simulink model "Boeing787_NewMission_ElectricalThermal"  (R2016a)
settings: Solver=ode23tb  SolverMode=SingleTasking  StartTime=0.0  StopTime=18000  RelTol=1e-3
InitFcn:
  | load('SampleOutput.mat')
  | 
  | load('SampleFuelBurn.mat')
StartFcn:
  | tic
StopFcn:
  | ttt = toc
  | tend = eval(get_param(bdroot,'StopTime'));
  | disp(['Total Simulation Time (s) = ' num2str(ttt) 's']);
  | RTR =  ttt/tend
  | disp(['Simulation Speed is ' num2str(tend/ttt) 'x faster than real-time']);
undefined symbols (not defined in the file): CurrentMission, FuelBurn, seed
libraries: PowerFlowLib x18, simulink x12, powerlib_meascontrol x1
(part 2 of 17)

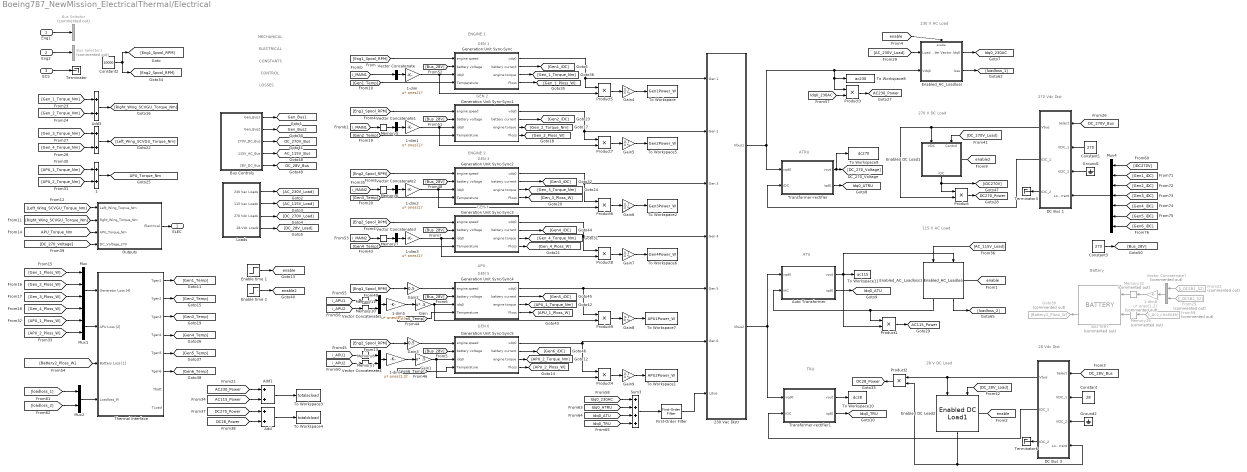
== system Boeing787_NewMission_ElectricalThermal/Electrical ==
  note: ATRU
  note: TRU
  note: 230 V AC Load
  note: 270 Vdc Dist
  note: 28 Vdc Dist
  note: 270 V DC Load
  note: CONSTANTS
  note: CONTROL
  note: LOSSES
  note: MECHANICAL
  note: ELECTRICAL
  note: ATU
  note: 115 V AC Load
  note: 28 V DC Load
  note: Battery
  note: GEN 1
  note: ENGINE 1
  note: GEN 2
  note: GEN 3
  note: ENGINE 2
  note: GEN 4
  note: GEN 5
  note: APU
  note: GEN 6
  Eng1 : Inport
  Eng2 : Inport  Port=2
  ECS : Inport  Port=3
  " " : Sum
  " 1" : Sum
  1-dim{,1..3} (4 alike) : Gain  Gain=ones(1)'  Multiplication=Matrix(u*K)
  1-dim4 : Gain  Gain=ones(1,2)'  Multiplication=Matrix(u*K)
  1-dim5 : Gain  Gain=ones(1,2)'  Multiplication=Matrix(u*K)
  1-dim8 : Gain  Commented=on  Gain=ones(1,2)'  Multiplication=Matrix(u*K)
  230 Vac Distr : Subsystem
  Add : Sum
  Add1 : Sum
  Add3 : Sum
  Auto Transformer : Subsystem  AncestorBlock=PowerFlowLib/Energy & Power Systems/Electrical/Systems/Transformer-rectifier  mask{pu=1}
      mask prompts: pu "Voltage Regulation Level (p.u.)"
      mask Display:
      | image('ATU.png')
      | % Define Inputs
      | port_label('input',1,'{\bf V_d_q_0}','Texmode','on')
      | port_label('input',2,'{\bf i_{dq0}}','Texmode','on')
      | 
      | % Define Outputs
      | port_label('output',1,'{\bf V_d_q_0}','Texmode','on')
      | port_label('output',2,'{\bf I_d_q_0}','Texmode','on')
      | 
      | 
      | % % Define Inputs
      | % port_label('input',1,'{\bf Line Voltage}','Texmode','on')
      | % port_label('input',2,'{\bf Line Voltage}','Texmode','on')
      | %
      | % % Define Outputs
      | % port_label('output',1,'{\bf Line Voltage}','Texmode','on')
      | % port_label('output',2,'{\bf Line Voltage}','Texmode','on')
  BATTERY : PowerFlowLib/Energy & Power Systems/Electrical/Battery/BATTERY  Commented=on  NO_CELLS=9  NO_MODULES=10  INITIAL_SOC=1
  Bus Selector : BusSelector  Commented=on  OutputSignals=Spools.HPSpoolSpeed_rpm
  Bus Selector1 : BusSelector  Commented=on  OutputSignals=Spools.HPSpoolSpeed_rpm
  Bus Controls : Subsystem  mask{BUS1=Generator 1, BUS2=Generator 2, MBUS1=Generator Bus 1, ACTBUS1=Generator Bus 1, MBUS2=Generator Bus 2, ACTBUS2=Generator Bus 2, IDCBUS1=Battery 1, IDCBUS2=Battery 2}
      mask prompts: BUS1 "Source for Bus 1"; BUS2 "Source for Bus 2"; MBUS1 "Load on Main Bus 1 drawn from"; ACTBUS1 "Load on AC Transfer Bus 1 drawn from"; MBUS2 "Load on Main Bus 2 drawn from"; ACTBUS2 "Load on AC Transfer Bus 2 drawn from"; IDCBUS1 "Source for DC Service Bus 1"; IDCBUS2 "Source for DC Service Bus 2"
      mask help:
      | Specify the source from which different buses receive power. There are
      | 1. Two Generator buses (Bus 1-2)
      | 2. Two AC Main buses (Main Bus 1-2))
      | 3. Two AC Transfer buses and (AC Transfer Bus 1-2)
      | 4. Two DC Intermediate buses (DC Intermediate Bus 1-2)
      mask init:
      | switch BUS1
      |     case 1
      |         BUS1CONTROL = 1;
      |     case 2
      |         BUS1CONTROL = 2;
      |     case 3
      |         BUS1CONTROL = 3;
      |     case 4
      |         BUS1CONTROL = 4;
      | end
      | 
      | switch BUS2
      |     case 1
      |         BUS2CONTROL = 1;
      |     case 2
      |         BUS2CONTROL = 2;
      |     case 3
      |         BUS2CONTROL = 3;
      |     case 4
      |         BUS2CONTROL = 4;
      | end
      | 
      | switch MBUS1
      |     case 1
      |         MBUS1CONTROL = 1;
      |     case 2
      |         MBUS1CONTROL = 2;
      | end
      | 
      | switch ACTBUS1
      |     case 1
      |         ACTBUS1CONTROL = 1;
      |     case 2
      |         ACTBUS1CONTROL = 2;
      | end
      | 
      | switch MBUS2
      |     case 1
      |         MBUS2CONTROL = 1;
      |     case 2
      |         MBUS2CONTROL = 2;
      | end
      | 
      | switch ACTBUS2
      |     case 1
      |         ACTBUS2CONTROL = 1;
      |     case 2
      |         ACTBUS2CONTROL = 2;
      | end
      | 
      | switch IDCBUS1
      |     case 1
      |         IDCBUS1CONTROL = 1;
      |     case 2
      |         IDCBUS1CONTROL = 2;
      | end
      | 
      | switch IDCBUS2
      |     case 1
      |         IDCBUS2CONTROL = 1;
      |     case 2
      |         IDCBUS2CONTROL = 2;
      | end
      mask TypeOptions BUS1: Generator 1  | APU  | GND | AUX SUPPLY
      mask TypeOptions BUS2: Generator 2  | APU  | GND | AUX SUPPLY
      mask TypeOptions MBUS1: Generator Bus 1 | Generator Bus 2
      mask TypeOptions ACTBUS1: Generator Bus 1 | Generator Bus 2
      mask TypeOptions MBUS2: Generator Bus 1 | Generator Bus 2
      mask TypeOptions ACTBUS2: Generator Bus 1 | Generator Bus 2
      mask TypeOptions IDCBUS1: Battery 1 | Battery 2
      mask TypeOptions IDCBUS2: Battery 1 | Battery 2
  Constant : Constant  Value=28
  Constant1 : Constant  Value=270
  Constant2 : Constant  Value=10000
  Constant3 : Constant  Value=270
  DC Bus 1 : Subsystem  mask(DC Service Bus){}
      mask help: Service Bus
  DC Bus 3 : Subsystem  mask(DC Service Bus){}
      mask help: Service Bus
  Enable time 1 : Step  Time=100  SampleTime=0
  Enable time 2 : Step  Time=105  SampleTime=0
  Enabled DC Load1 : Subsystem  AncestorBlock="PowerFlowLib/Energy & Power Systems/Electrical/Loads/Enabled  DC Load1"
      mask help: Enabled DC Load System.
      mask Display:
      | image(imread('DCloads.png'))
      | 
      | port_label('input',1,'{\bf V_D_C}','TexMode','on')
      | port_label('input',2,'{\bf Load}','TexMode','on')
      | port_label('Enable','{\bf switch}','Texmode','on')
      | 
      | port_label('output',1,'{\bf I_D_C}','TexMode','on')
  Enabled DC Load2 : PowerFlowLib/Energy & Power Systems/Electrical/Loads/Enabled  DC Load1
  Enabled_AC_Loadloss : Subsystem  AncestorBlock=PowerFlowLib/Energy & Power Systems/Electrical/Loads/Enabled_AC_Loadloss  mask(AC Loads){P=500, PF=0.85, ILRMS=0, R=10000, X=10000}
      mask prompts: P "Real Power (W)"; PF "Power factor (Range: 0 -1) : Prefix '-' sign for Cap loads"; ILRMS "Current Loading"; R "Resistance (Ohms)"; X "Reactance (Ohms)"
      mask help:
      | Enabled AC Load System.
      | Note:
      | Load Master Vector input is 1x3 matrix representing (P[W] Q[Var] I[A])
      | Extra load can be input in the boxes below and will be added with the Load Master Vector.
      mask Help: eval('open(''AC Loads_help.html'')');
      mask Callback PF:
      | blk = gcb;
      | PF    = str2num(get_param(blk,'PF'));
      | 
      | if ((PF>1) | (PF<-1))
      |    g = warndlg('Power factor magnitude should be between 0 and 1 . Reverting to default value 1','Error1','CreateMode');
      |    set_param(blk,'PF','1');
      |    open_system(blk,'mask');
      | end
      | 
      | clear g PF blk
      mask Callback X:
      | blk = gcb;
      | value1 = str2num(get_param(blk,'R'));
      | value2 = str2num(get_param(blk,'X'));
      | % eff    = str2num(get_param(blk,'E'));
      | 
      | if (value1==0) && (value2==0)
      |   h = warndlg('Both R and X cannot be 0. Reverting to default values','Error','CreateMode');
      |   set_param(blk,'R','10000');
      |   set_param(blk,'X','10000');
      | %   if ishandle(h)
      | %       close(h)
      |   open_system(blk,'mask');
      | end
      | 
      | % if ((eff>1) | (eff<0))
      | %    g = warndlg('Efficiency should be between 0 and 1 . Reverting to default value 1','Error1','CreateMode');
      | %    set_param(blk,'E','1');
      | %    open_system(blk,'mask');
      | % end
      | 
      | clear h eff blk value1 value2
      mask Display:
      | %image(imread('ACload.png'))
      | 
      | % port_label('input',1,'{\bf EXT LOAD VECTOR}','TexMode','on')
      | % port_label('input',2,'{\bf Vdq0}','TexMode','on')
      | %
      | % port_label('output',1,'{\bf Idq0}','TexMode','on')
      | % port_label('output',2,'{\bf PLOSS}','TexMode','on')
      | 
      | image(imread('ACloads.png'))
      | 
      | port_label('input',1,'{\bf Load}','TexMode','on')
      | port_label('input',2,'{\bf V_d_q_0}','TexMode','on')
      | port_label('Enable','{\bf switch}','Texmode','on')
      | 
      | port_label('output',1,'{\bf I_d_q_0}','TexMode','on')
      | port_label('output',2,'{\bf P_l_o_s_s}','TexMode','on')
  Enabled_AC_Loadloss1 : PowerFlowLib/Energy & Power Systems/Electrical/Loads/Enabled_AC_Loadloss  P=500  PF=0.85  ILRMS=0  R=10000  X=10000
  First-Order Filter : powerlib_meascontrol/Filters/First-Order Filter  FilterType=Lowpass  Tc=10e-1  Ts=0  Initialize=on  Vac_Init=[0, 0, 60]  Vdc_Init=0  PlotResponse=off  FreqRange="[0,  200,  1]"
  From22 : From  Commented=on  GotoTag=i_DCSB1_S2
  From25 : From  Commented=on  GotoTag=i_DCSB2_S2
  From59 : From  Commented=on  GotoTag=i_DC2_CHARGER
  Gain : Gain  Gain=.5  Multiplication=Matrix(u*K)
  Gain1 : Gain  Gain=.5  Multiplication=Matrix(u*K)
  Gain2 : Gain  Gain=0.5
  Gain3 : Gain  Gain=0.5
  Gain{4..9} (6 alike) : Gain  Gain=[1 1 1]  Multiplication=Matrix(K*u) (u vector)
  Generation Unit Sync-Sync : Subsystem  AncestorBlock=PowerFlowLib/Energy & Power Systems/Electrical/Systems/Generation Unit Sync-Sync  mask{machine_mode=300kVA_Gen, Rs=0.007845, Xls=0.0030003, Xmd=0.83467, Xmq=0.0009001, R_fd=0.0024787, Xlfd=0.12144, R_1d=0.072117, Xl1d=0.60648, R_1q=0.019173, R_2q=0.019173, Xl1q=0.10831, Xl2q=0.10831, ws=377, RTL=0.001, XTL=0.1, KA=20, KF=0.063, T_f=0.35, TA=0.2, KE=1, TE=0.314, SB=300000, VBDQ=100, wB=377, P=2, H=0.17945, R_conv_gen=0.05, mc_gen=10000, Vnom=230, fan_load='init_fan_characteristics.mat', exciter_param='exciter.mat'}
      mask prompts: machine_mode "Machine Preset"; Rs "Stator Resistance [ohm]"; Xls "Stator Leakage Reactance [ohm]"; Xmd "Magnetizing Direct Axis Reactance [ohm]"; Xmq "Magnetizing Quadrature Axis Reactance [ohm]"; R_fd "Field Resistance [ohm]"; Xlfd "Field Leakage Reactance [ohm]"; R_1d "Transient Direct Axis Resistance [ohm]"; Xl1d "Transient Leakage Direct Axis Reactance [ohm]"; R_1q "Transient Quadrature Axis Resistance [ohm]"; R_2q "Subtransient Quadrature Axis Resistance [ohm]"; Xl1q "Transient Leakage Quadrature Axis Reactance [ohm]"; Xl2q "Subtransient Leakage Quadrature Axis Reactance [ohm]"; ws "Rotational Speed [rad/s]"; RTL "Resistance [ohm]"; XTL "Reactance [ohm]"; SB "Baes Complex Power [VA]"; VBDQ "Base Direct and Quadrature Axis Armature Voltage [V]"; wB "Base Electrical Frequency [rad/s]"; P "Number of Pole Pairs"; H "Shaft Inertia Constant [s]"; Vnom "Nominal Voltage [V]"; fan_load "Fan Load"; exciter_param "Exciter Machine Parameters"
      mask help:
      | A generator system block implements a generic power generation unit consisting of a gearbox, a synchronous generator, a synchronous exciter and exciter controls.
      | The generator size can be selected from the drop window below.
      | (For advanced-users) When the User-defined option is selected from the drop window, the generator parameters can be manually specified in the tabs below.
      |
      | Block Inputs:
      |
      | #1: Jet engine low pressure spool [RPM]
      | #2: Exciter system supply voltage [V]
      | #3: Synchronous reference frame line currents  [A]
      |
      | Block Output:
      |
      | #1: Synchronous reference frame line voltages [V]
      | #2: Exciter system supply current [A]
      | #3: Electromagnetic torque on the low pressure spool  [N-M]
      | #4: Heat rejected to the cooling system or ambient [W]
      mask init:
      | load(fan_load);
      | 
      | % Inductances
      | Xd = Xls + Xmd;
      | Xq = Xls + Xmq;
      | Xfd = Xlfd + Xmd;
      | X1q = Xl1q + Xmq;
      | Xd1 = Xd - Xmd^2/Xfd;
      | Xq1 = Xq - Xmq^2/X1q;
      | Xd2 = Xls + (1/(1/Xmd + 1/Xlfd + 1/Xl1d));
      | Xq2 = Xls + (1/(1/Xmq + 1/Xl1q + 1/Xl2q));
      | Tdo1 = Xfd/ws/R_fd;
      | Tqo1 = X1q/ws/R_1q;
      | Tdo2 = 1/ws/R_1d*(Xl1d + 1/(1/Xmd + 1/Xlfd));
      | Tqo2 = 1/ws/R_2q*(Xl2q+1/(1/Xmq + 1/Xl1q));
      | 
      | % Base Quantities
      | 
      | TB = (P/2)*SB/wB;
      | IBDQ = SB/VBDQ;
      | LBDQ = VBDQ/wB;
      | 
      | IBFD = IBDQ;
      | IB1D = IBDQ;
      | IB1Q = IBDQ;
      | IB2Q = IBDQ;
      | 
      | VBFD = SB/IBFD;
      | VB1D = SB/IB1D;
      | VB1Q = SB/IB1Q;
      | VB2Q = SB/IB2Q;
      | 
      | LBFD = VBFD/wB;
      | LB1D = VB1D/wB;
      | LB1Q = VB1Q/wB;
      | LB2Q = VB2Q/wB;
      | 
      | J = 2*H/(wB*2/P)^2*SB;
      | M = 2*H/wB;
      | 
      | % Exciter
      | 
      | data_exc = load(exciter_param);
      |   
      | % Stator
      | Rs_exc = data_exc.r(1);
      | Xls_exc = data_exc.r(2);
      | Xmd_exc = data_exc.r(3);
      | Xmq_exc = data_exc.r(4);
      | 
      | % Field
      | R_fd_exc = data_exc.r(5);
      | Xlfd_exc = data_exc.r(6);
      | % Dampers
      | R_1d_exc = data_exc.r(7);
      | Xl1d_exc = data_exc.r(8);
      | R_1q_exc = data_exc.r(9);
      | Xl1q_exc = data_exc.r(10);
      | R_2q_exc = data_exc.r(11);
      | Xl2q_exc = data_exc.r(12);
      | 
      | % Rotor
      | P_exc = data_exc.r(13);
      | ws_exc = data_exc.r(14);
      | 
      | % Inductances
      | Xd_exc = Xls_exc + Xmd_exc;
      | Xq_exc = Xls_exc + Xmq_exc;
      | Xfd_exc = Xlfd_exc + Xmd_exc;
      | X1q_exc = Xl1q_exc + Xmq_exc;
      | Xd1_exc = Xd_exc - Xmd_exc^2/Xfd_exc;
      | Xq1_exc = Xq_exc - Xmq_exc^2/X1q_exc;
      | Xd2_exc = Xls_exc + (1/(1/Xmd_exc + 1/Xlfd_exc + 1/Xl1d_exc));
      | Xq2_exc = Xls_exc + (1/(1/Xmq_exc + 1/Xl1q_exc + 1/Xl2q_exc));
      | Tdo1_exc = Xfd_exc/ws_exc/R_fd_exc;
      | Tqo1_exc = X1q_exc/ws_exc/R_1q_exc;
      | Tdo2_exc = 1/ws_exc/R_1d_exc*(Xl1d_exc + 1/(1/Xmd_exc + 1/Xlfd_exc));
      | Tqo2_exc = 1/ws_exc/R_2q_exc*(Xl2q_exc+1/(1/Xmq_exc + 1/Xl1q_exc));
      | 
      | % Transmission Line
      | RTL_exc = data_exc.r(15);
      | XTL_exc = data_exc.r(16);
      | 
      | % Regulator and Governor
      | KA_exc = data_exc.r(17);
      | KF_exc = data_exc.r(18);
      | T_f_exc = data_exc.r(19);
      | TA_exc = data_exc.r(20);
      | KE_exc = data_exc.r(21);
      | TE_exc = data_exc.r(22);
      | 
      | % Base Quantities
      | SB_exc = data_exc.r(23);
      | VBDQ_exc = data_exc.r(24);
      | wB_exc = data_exc.r(25);
      | P_exc = data_exc.r(13);
      | H_exc = data_exc.r(26);
      | 
      | TB_exc = (P/2)*SB_exc/wB_exc;
      | IBDQ_exc = SB_exc/VBDQ_exc;
      | LBDQ_exc = VBDQ_exc/wB_exc;
      | 
      | IBFD_exc = IBDQ_exc;
      | IB1D_exc = IBDQ_exc;
      | IB1Q_exc = IBDQ_exc;
      | IB2Q_exc = IBDQ_exc;
      | 
      | VBFD_exc = SB_exc/IBFD_exc;
      | VB1D_exc = SB_exc/IB1D_exc;
      | VB1Q_exc = SB_exc/IB1Q_exc;
      | VB2Q_exc = SB_exc/IB2Q_exc;
      | 
      | LBFD_exc = VBFD_exc/wB_exc;
      | LB1D_exc = VB1D_exc/wB_exc;
      | LB1Q_exc = VB1Q_exc/wB_exc;
      | LB2Q_exc = VB2Q_exc/wB_exc;
      | 
      | J_exc = 2*data_exc.r(26)/(wB_exc*2/P_exc)^2*SB_exc;
      | M_exc = 2*H_exc/wB_exc;
      | 
      | R_conv_gen_exc = 1/data_exc.r(27);
      | mc_gen_exc = data_exc.r(28);
      mask Help: eval('open(''Generator System_help.html'')');
      mask TypeOptions machine_mode: 20kVA_Gen | 52.5kVA_Gen | 100kVA_Gen | 300kVA_Gen | 800kVA_Gen | 1MVA_Gen | User-defined
      mask Callback machine_mode:
      | h=get_param(gcb,'handle');
      | hblock=get(h);
      | data=load('GenProp.mat');
      | 
      | if strcmp(hblock.machine_mode,'User-defined')==1;
      |     adv_warn=warndlg(sprintf('User-defined parameters may lead to an unstable build.'));
      | 
      |     % grabs current values of enabled GUI parameters
      |     mskenabl = get_param(gcb,'MaskEnables');
      |     mskenabl(1:size(mskenabl,1)) = {'on'};  % sets all parameters to enable
      |     set_param(gcb,'MaskEnables',mskenabl)
      | 
      | else
      |     % For each generator preset references a column from GenProp.mat
      |     if strcmp(hblock.machine_mode,'20kVA_Gen')==1; n=1;
      |     elseif strcmp(hblock.machine_mode,'52.5kVA_Gen')==1; n=2;
      |     elseif strcmp(hblock.machine_mode,'100kVA_Gen')==1; n=3;
      |     elseif strcmp(hblock.machine_mode,'300kVA_Gen')==1; n=4;
      |     elseif strcmp(hblock.machine_mode,'800kVA_Gen')==1; n=5;
      |     elseif strcmp(hblock.machine_mode,'1MVA_Gen')==1; n=6;
      |     end
      |     % Set each parameter of the generator
      |     set1=num2str(data.r(1,n));
      |     set2=num2str(data.r(2,n));
      |     set3=num2str(data.r(3,n));
      |     set4=num2str(data.r(4,n));
      |     set_param(gcb,'Rs',set1,'Xls',set2,'Xmd',set3,'Xmq',set4)
      |     set1=num2str(data.r(5,n));
      |     set2=num2str(data.r(6,n));
      |     set_param(gcb,'R_fd',set1,'Xlfd',set2) %5 and 6
      |     set1=num2str(data.r(7,n));
      |     set2=num2str(data.r(8,n));
      |     set3=num2str(data.r(9,n));
      |     set4=num2str(data.r(10,n));
      |     set5=num2str(data.r(11,n));
      |     set6=num2str(data.r(12,n));
      |     set_param(gcb,'R_1d',set1,'Xl1d',set2,'R_1q',set3,'Xl1q',set4,'R_2q',set5,'Xl2q',set6) %7-12
      |     set1=num2str(data.r(14,n));
      |     set2=num2str(data.r(15,n));
      |     set3=num2str(data.r(16,n));
      |     set_param(gcb,'ws',set1,'RTL',set2,'XTL',set3)
      |     set1=num2str(data.r(17,n));
      |     set2=num2str(data.r(18,n));
      |     set3=num2str(data.r(19,n));
      |     set4=num2str(data.r(20,n));
      |     set5=num2str(data.r(21,n));
      |     set6=num2str(data.r(22,n));
      |     set_param(gcb,'KA',set1,'KF',set2,'T_f',set3,'TA',set4,'KE',set5,'TE',set6)
      |     set1=num2str(data.r(23,n));
      |     set2=num2str(data.r(24,n));
      |     set3=num2str(data.r(25,n));
      |     set4=num2str(data.r(13,n));
      |     set5=num2str(data.r(26,n));
      |     set_param(gcb,'SB',set1,'VBDQ',set2,'wB',set3,'P',set4,'H',set5)
      |     set1=num2str(1/data.r(27,n));
      |     set2=num2str(data.r(28,n));
      |     set_param(gcb,'R_conv_gen',set1,'mc_gen',set2)
      | 
      |     % grabs current values of enabled GUI parameters
      |     mskenabl = get_param(gcb,'MaskEnables');
      |     % sets all parameters to enable
      |     mskenabl(2:size(mskenabl,1)-3) = {'off'};
      |     set_param(gcb,'MaskEnables',mskenabl)
      | 
      | 
      | end
      | 
      | 
      | clear h hblock n data mskenabl
      | clear set1 set2 set3 set4 set5 set6
      mask Display:
      | image(imread('Generator.png')) % Load image
      | 
      | % Define inputs
      | 
      | port_label('input',1,'{\bf \omega_s_h_a_f_t}','Texmode','on')
      | port_label('input',2,'{\bf V_D_C}','Texmode','on')
      | port_label('input',3,'{\bf I_d_q_0}','Texmode','on')
      | port_label('input',4,'{\bf Temp}','Texmode','on')
      | 
      | % Define outputs
      | 
      | port_label('output',1,'{\bf V_d_q_0}','Texmode','on')
      | port_label('output',2,'{\bf I_D_C}','Texmode','on')
      | port_label('output',3,'{\bf \tau}','Texmode','on')
      | port_label('output',4,'{\bf P_l_o_s_s}','Texmode','on')
      | 
      | % % Define inputs
      | %
      | % port_label('input',1,'{\bf Generator Speed}','Texmode','on')
      | % port_label('input',2,'{\bf Battery Voltage}','Texmode','on')
      | % port_label('input',3,'{\bf Line Currents}','Texmode','on')
      | %
      | % % Define outputs
      | %
      | % port_label('output',1,'{\bf Line Voltages}','Texmode','on')
      | % port_label('output',2,'{\bf Battery Current}','Texmode','on')
      | % port_label('output',3,'{\bf Generator Torque}','Texmode','on')
      | % port_label('output',4,'{\bf Power Loss}','Texmode','on')
  Generation Unit Sync-Sync1 : Subsystem  AncestorBlock=PowerFlowLib/Energy & Power Systems/Electrical/Systems/Generation Unit Sync-Sync  mask{machine_mode=300kVA_Gen, Rs=0.007845, Xls=0.0030003, Xmd=0.83467, Xmq=0.0009001, R_fd=0.0024787, Xlfd=0.12144, R_1d=0.072117, Xl1d=0.60648, R_1q=0.019173, R_2q=0.019173, Xl1q=0.10831, Xl2q=0.10831, ws=377, RTL=0.001, XTL=0.1, KA=20, KF=0.063, T_f=0.35, TA=0.2, KE=1, TE=0.314, SB=300000, VBDQ=100, wB=377, P=2, H=0.17945, R_conv_gen=0.05, mc_gen=10000, Vnom=230, fan_load='init_fan_characteristics.mat', exciter_param='exciter.mat'}
      mask prompts: machine_mode "Machine Preset"; Rs "Stator Resistance [ohm]"; Xls "Stator Leakage Reactance [ohm]"; Xmd "Magnetizing Direct Axis Reactance [ohm]"; Xmq "Magnetizing Quadrature Axis Reactance [ohm]"; R_fd "Field Resistance [ohm]"; Xlfd "Field Leakage Reactance [ohm]"; R_1d "Transient Direct Axis Resistance [ohm]"; Xl1d "Transient Leakage Direct Axis Reactance [ohm]"; R_1q "Transient Quadrature Axis Resistance [ohm]"; R_2q "Subtransient Quadrature Axis Resistance [ohm]"; Xl1q "Transient Leakage Quadrature Axis Reactance [ohm]"; Xl2q "Subtransient Leakage Quadrature Axis Reactance [ohm]"; ws "Rotational Speed [rad/s]"; RTL "Resistance [ohm]"; XTL "Reactance [ohm]"; SB "Baes Complex Power [VA]"; VBDQ "Base Direct and Quadrature Axis Armature Voltage [V]"; wB "Base Electrical Frequency [rad/s]"; P "Number of Pole Pairs"; H "Shaft Inertia Constant [s]"; Vnom "Nominal Voltage [V]"; fan_load "Fan Load"; exciter_param "Exciter Machine Parameters"
      mask help:
      | A generator system block implements a generic power generation unit consisting of a gearbox, a synchronous generator, a synchronous exciter and exciter controls.
      | The generator size can be selected from the drop window below.
      | (For advanced-users) When the User-defined option is selected from the drop window, the generator parameters can be manually specified in the tabs below.
      |
      | Block Inputs:
      |
      | #1: Jet engine low pressure spool [RPM]
      | #2: Exciter system supply voltage [V]
      | #3: Synchronous reference frame line currents  [A]
      |
      | Block Output:
      |
      | #1: Synchronous reference frame line voltages [V]
      | #2: Exciter system supply current [A]
      | #3: Electromagnetic torque on the low pressure spool  [N-M]
      | #4: Heat rejected to the cooling system or ambient [W]
      mask init: same as Boeing787_NewMission_ElectricalThermal/Electrical/Generation Unit Sync-Sync
      mask Help: eval('open(''Generator System_help.html'')');
      mask TypeOptions machine_mode: 20kVA_Gen | 52.5kVA_Gen | 100kVA_Gen | 300kVA_Gen | 800kVA_Gen | 1MVA_Gen | User-defined
      mask Callback machine_mode:
      | h=get_param(gcb,'handle');
      | hblock=get(h);
      | data=load('GenProp.mat');
      | 
      | if strcmp(hblock.machine_mode,'User-defined')==1;
      |     adv_warn=warndlg(sprintf('User-defined parameters may lead to an unstable build.'));
      | 
      |     % grabs current values of enabled GUI parameters
      |     mskenabl = get_param(gcb,'MaskEnables');
      |     mskenabl(1:size(mskenabl,1)) = {'on'};  % sets all parameters to enable
      |     set_param(gcb,'MaskEnables',mskenabl)
      | 
      | else
      |     % For each generator preset references a column from GenProp.mat
      |     if strcmp(hblock.machine_mode,'20kVA_Gen')==1; n=1;
      |     elseif strcmp(hblock.machine_mode,'52.5kVA_Gen')==1; n=2;
      |     elseif strcmp(hblock.machine_mode,'100kVA_Gen')==1; n=3;
      |     elseif strcmp(hblock.machine_mode,'300kVA_Gen')==1; n=4;
      |     elseif strcmp(hblock.machine_mode,'800kVA_Gen')==1; n=5;
      |     elseif strcmp(hblock.machine_mode,'1MVA_Gen')==1; n=6;
      |     end
      |     % Set each parameter of the generator
      |     set1=num2str(data.r(1,n));
      |     set2=num2str(data.r(2,n));
      |     set3=num2str(data.r(3,n));
      |     set4=num2str(data.r(4,n));
      |     set_param(gcb,'Rs',set1,'Xls',set2,'Xmd',set3,'Xmq',set4)
      |     set1=num2str(data.r(5,n));
      |     set2=num2str(data.r(6,n));
      |     set_param(gcb,'R_fd',set1,'Xlfd',set2) %5 and 6
      |     set1=num2str(data.r(7,n));
      |     set2=num2str(data.r(8,n));
      |     set3=num2str(data.r(9,n));
      |     set4=num2str(data.r(10,n));
      |     set5=num2str(data.r(11,n));
      |     set6=num2str(data.r(12,n));
      |     set_param(gcb,'R_1d',set1,'Xl1d',set2,'R_1q',set3,'Xl1q',set4,'R_2q',set5,'Xl2q',set6) %7-12
      |     set1=num2str(data.r(14,n));
      |     set2=num2str(data.r(15,n));
      |     set3=num2str(data.r(16,n));
      |     set_param(gcb,'ws',set1,'RTL',set2,'XTL',set3)
      |     set1=num2str(data.r(17,n));
      |     set2=num2str(data.r(18,n));
      |     set3=num2str(data.r(19,n));
      |     set4=num2str(data.r(20,n));
      |     set5=num2str(data.r(21,n));
      |     set6=num2str(data.r(22,n));
      |     set_param(gcb,'KA',set1,'KF',set2,'T_f',set3,'TA',set4,'KE',set5,'TE',set6)
      |     set1=num2str(data.r(23,n));
      |     set2=num2str(data.r(24,n));
      |     set3=num2str(data.r(25,n));
      |     set4=num2str(data.r(13,n));
      |     set5=num2str(data.r(26,n));
      |     set_param(gcb,'SB',set1,'VBDQ',set2,'wB',set3,'P',set4,'H',set5)
      |     set1=num2str(1/data.r(27,n));
      |     set2=num2str(data.r(28,n));
      |     set_param(gcb,'R_conv_gen',set1,'mc_gen',set2)
      | 
      |     % grabs current values of enabled GUI parameters
      |     mskenabl = get_param(gcb,'MaskEnables');
      |     % sets all parameters to enable
      |     mskenabl(2:size(mskenabl,1)-3) = {'off'};
      |     set_param(gcb,'MaskEnables',mskenabl)
      | 
      | 
      | end
      | 
      | 
      | clear h hblock n data mskenabl
      | clear set1 set2 set3 set4 set5 set6
      mask Display:
      | image(imread('Generator.png')) % Load image
      | 
      | % Define inputs
      | 
      | port_label('input',1,'{\bf \omega_s_h_a_f_t}','Texmode','on')
      | port_label('input',2,'{\bf V_D_C}','Texmode','on')
      | port_label('input',3,'{\bf I_d_q_0}','Texmode','on')
      | port_label('input',4,'{\bf Temp}','Texmode','on')
      | 
      | % Define outputs
      | 
      | port_label('output',1,'{\bf V_d_q_0}','Texmode','on')
      | port_label('output',2,'{\bf I_D_C}','Texmode','on')
      | port_label('output',3,'{\bf \tau}','Texmode','on')
      | port_label('output',4,'{\bf P_l_o_s_s}','Texmode','on')
      | 
      | % % Define inputs
      | %
      | % port_label('input',1,'{\bf Generator Speed}','Texmode','on')
      | % port_label('input',2,'{\bf Battery Voltage}','Texmode','on')
      | % port_label('input',3,'{\bf Line Currents}','Texmode','on')
      | %
      | % % Define outputs
      | %
      | % port_label('output',1,'{\bf Line Voltages}','Texmode','on')
      | % port_label('output',2,'{\bf Battery Current}','Texmode','on')
      | % port_label('output',3,'{\bf Generator Torque}','Texmode','on')
      | % port_label('output',4,'{\bf Power Loss}','Texmode','on')
  Generation Unit Sync-Sync2 : Subsystem  AncestorBlock=PowerFlowLib/Energy & Power Systems/Electrical/Systems/Generation Unit Sync-Sync  mask{machine_mode=300kVA_Gen, Rs=0.007845, Xls=0.0030003, Xmd=0.83467, Xmq=0.0009001, R_fd=0.0024787, Xlfd=0.12144, R_1d=0.072117, Xl1d=0.60648, R_1q=0.019173, R_2q=0.019173, Xl1q=0.10831, Xl2q=0.10831, ws=377, RTL=0.001, XTL=0.1, KA=20, KF=0.063, T_f=0.35, TA=0.2, KE=1, TE=0.314, SB=300000, VBDQ=100, wB=377, P=2, H=0.17945, R_conv_gen=0.05, mc_gen=10000, Vnom=230, fan_load='init_fan_characteristics.mat', exciter_param='exciter.mat'}
      mask prompts: machine_mode "Machine Preset"; Rs "Stator Resistance [ohm]"; Xls "Stator Leakage Reactance [ohm]"; Xmd "Magnetizing Direct Axis Reactance [ohm]"; Xmq "Magnetizing Quadrature Axis Reactance [ohm]"; R_fd "Field Resistance [ohm]"; Xlfd "Field Leakage Reactance [ohm]"; R_1d "Transient Direct Axis Resistance [ohm]"; Xl1d "Transient Leakage Direct Axis Reactance [ohm]"; R_1q "Transient Quadrature Axis Resistance [ohm]"; R_2q "Subtransient Quadrature Axis Resistance [ohm]"; Xl1q "Transient Leakage Quadrature Axis Reactance [ohm]"; Xl2q "Subtransient Leakage Quadrature Axis Reactance [ohm]"; ws "Rotational Speed [rad/s]"; RTL "Resistance [ohm]"; XTL "Reactance [ohm]"; SB "Baes Complex Power [VA]"; VBDQ "Base Direct and Quadrature Axis Armature Voltage [V]"; wB "Base Electrical Frequency [rad/s]"; P "Number of Pole Pairs"; H "Shaft Inertia Constant [s]"; Vnom "Nominal Voltage [V]"; fan_load "Fan Load"; exciter_param "Exciter Machine Parameters"
      mask help:
      | A generator system block implements a generic power generation unit consisting of a gearbox, a synchronous generator, a synchronous exciter and exciter controls.
      | The generator size can be selected from the drop window below.
      | (For advanced-users) When the User-defined option is selected from the drop window, the generator parameters can be manually specified in the tabs below.
      |
      | Block Inputs:
      |
      | #1: Jet engine low pressure spool [RPM]
      | #2: Exciter system supply voltage [V]
      | #3: Synchronous reference frame line currents  [A]
      |
      | Block Output:
      |
      | #1: Synchronous reference frame line voltages [V]
      | #2: Exciter system supply current [A]
      | #3: Electromagnetic torque on the low pressure spool  [N-M]
      | #4: Heat rejected to the cooling system or ambient [W]
      mask init: same as Boeing787_NewMission_ElectricalThermal/Electrical/Generation Unit Sync-Sync
      mask Help: eval('open(''Generator System_help.html'')');
      mask TypeOptions machine_mode: 20kVA_Gen | 52.5kVA_Gen | 100kVA_Gen | 300kVA_Gen | 800kVA_Gen | 1MVA_Gen | User-defined
      mask Callback machine_mode:
      | h=get_param(gcb,'handle');
      | hblock=get(h);
      | data=load('GenProp.mat');
      | 
      | if strcmp(hblock.machine_mode,'User-defined')==1;
      |     adv_warn=warndlg(sprintf('User-defined parameters may lead to an unstable build.'));
      | 
      |     % grabs current values of enabled GUI parameters
      |     mskenabl = get_param(gcb,'MaskEnables');
      |     mskenabl(1:size(mskenabl,1)) = {'on'};  % sets all parameters to enable
      |     set_param(gcb,'MaskEnables',mskenabl)
      | 
      | else
      |     % For each generator preset references a column from GenProp.mat
      |     if strcmp(hblock.machine_mode,'20kVA_Gen')==1; n=1;
      |     elseif strcmp(hblock.machine_mode,'52.5kVA_Gen')==1; n=2;
      |     elseif strcmp(hblock.machine_mode,'100kVA_Gen')==1; n=3;
      |     elseif strcmp(hblock.machine_mode,'300kVA_Gen')==1; n=4;
      |     elseif strcmp(hblock.machine_mode,'800kVA_Gen')==1; n=5;
      |     elseif strcmp(hblock.machine_mode,'1MVA_Gen')==1; n=6;
      |     end
      |     % Set each parameter of the generator
      |     set1=num2str(data.r(1,n));
      |     set2=num2str(data.r(2,n));
      |     set3=num2str(data.r(3,n));
      |     set4=num2str(data.r(4,n));
      |     set_param(gcb,'Rs',set1,'Xls',set2,'Xmd',set3,'Xmq',set4)
      |     set1=num2str(data.r(5,n));
      |     set2=num2str(data.r(6,n));
      |     set_param(gcb,'R_fd',set1,'Xlfd',set2) %5 and 6
      |     set1=num2str(data.r(7,n));
      |     set2=num2str(data.r(8,n));
      |     set3=num2str(data.r(9,n));
      |     set4=num2str(data.r(10,n));
      |     set5=num2str(data.r(11,n));
      |     set6=num2str(data.r(12,n));
      |     set_param(gcb,'R_1d',set1,'Xl1d',set2,'R_1q',set3,'Xl1q',set4,'R_2q',set5,'Xl2q',set6) %7-12
      |     set1=num2str(data.r(14,n));
      |     set2=num2str(data.r(15,n));
      |     set3=num2str(data.r(16,n));
      |     set_param(gcb,'ws',set1,'RTL',set2,'XTL',set3)
      |     set1=num2str(data.r(17,n));
      |     set2=num2str(data.r(18,n));
      |     set3=num2str(data.r(19,n));
      |     set4=num2str(data.r(20,n));
      |     set5=num2str(data.r(21,n));
      |     set6=num2str(data.r(22,n));
      |     set_param(gcb,'KA',set1,'KF',set2,'T_f',set3,'TA',set4,'KE',set5,'TE',set6)
      |     set1=num2str(data.r(23,n));
      |     set2=num2str(data.r(24,n));
      |     set3=num2str(data.r(25,n));
      |     set4=num2str(data.r(13,n));
      |     set5=num2str(data.r(26,n));
      |     set_param(gcb,'SB',set1,'VBDQ',set2,'wB',set3,'P',set4,'H',set5)
      |     set1=num2str(1/data.r(27,n));
      |     set2=num2str(data.r(28,n));
      |     set_param(gcb,'R_conv_gen',set1,'mc_gen',set2)
      | 
      |     % grabs current values of enabled GUI parameters
      |     mskenabl = get_param(gcb,'MaskEnables');
      |     % sets all parameters to enable
      |     mskenabl(2:size(mskenabl,1)-3) = {'off'};
      |     set_param(gcb,'MaskEnables',mskenabl)
      | 
      | 
      | end
      | 
      | 
      | clear h hblock n data mskenabl
      | clear set1 set2 set3 set4 set5 set6
      mask Display:
      | image(imread('Generator.png')) % Load image
      | 
      | % Define inputs
      | 
      | port_label('input',1,'{\bf \omega_s_h_a_f_t}','Texmode','on')
      | port_label('input',2,'{\bf V_D_C}','Texmode','on')
      | port_label('input',3,'{\bf I_d_q_0}','Texmode','on')
      | port_label('input',4,'{\bf Temp}','Texmode','on')
      | 
      | % Define outputs
      | 
      | port_label('output',1,'{\bf V_d_q_0}','Texmode','on')
      | port_label('output',2,'{\bf I_D_C}','Texmode','on')
      | port_label('output',3,'{\bf \tau}','Texmode','on')
      | port_label('output',4,'{\bf P_l_o_s_s}','Texmode','on')
      | 
      | % % Define inputs
      | %
      | % port_label('input',1,'{\bf Generator Speed}','Texmode','on')
      | % port_label('input',2,'{\bf Battery Voltage}','Texmode','on')
      | % port_label('input',3,'{\bf Line Currents}','Texmode','on')
      | %
      | % % Define outputs
      | %
      | % port_label('output',1,'{\bf Line Voltages}','Texmode','on')
      | % port_label('output',2,'{\bf Battery Current}','Texmode','on')
      | % port_label('output',3,'{\bf Generator Torque}','Texmode','on')
      | % port_label('output',4,'{\bf Power Loss}','Texmode','on')
  Generation Unit Sync-Sync3 : Subsystem  AncestorBlock=PowerFlowLib/Energy & Power Systems/Electrical/Systems/Generation Unit Sync-Sync  mask{machine_mode=300kVA_Gen, Rs=0.007845, Xls=0.0030003, Xmd=0.83467, Xmq=0.0009001, R_fd=0.0024787, Xlfd=0.12144, R_1d=0.072117, Xl1d=0.60648, R_1q=0.019173, R_2q=0.019173, Xl1q=0.10831, Xl2q=0.10831, ws=377, RTL=0.001, XTL=0.1, KA=20, KF=0.063, T_f=0.35, TA=0.2, KE=1, TE=0.314, SB=300000, VBDQ=100, wB=377, P=2, H=0.17945, R_conv_gen=0.05, mc_gen=10000, Vnom=230, fan_load='init_fan_characteristics.mat', exciter_param='exciter.mat'}
      mask prompts: machine_mode "Machine Preset"; Rs "Stator Resistance [ohm]"; Xls "Stator Leakage Reactance [ohm]"; Xmd "Magnetizing Direct Axis Reactance [ohm]"; Xmq "Magnetizing Quadrature Axis Reactance [ohm]"; R_fd "Field Resistance [ohm]"; Xlfd "Field Leakage Reactance [ohm]"; R_1d "Transient Direct Axis Resistance [ohm]"; Xl1d "Transient Leakage Direct Axis Reactance [ohm]"; R_1q "Transient Quadrature Axis Resistance [ohm]"; R_2q "Subtransient Quadrature Axis Resistance [ohm]"; Xl1q "Transient Leakage Quadrature Axis Reactance [ohm]"; Xl2q "Subtransient Leakage Quadrature Axis Reactance [ohm]"; ws "Rotational Speed [rad/s]"; RTL "Resistance [ohm]"; XTL "Reactance [ohm]"; SB "Baes Complex Power [VA]"; VBDQ "Base Direct and Quadrature Axis Armature Voltage [V]"; wB "Base Electrical Frequency [rad/s]"; P "Number of Pole Pairs"; H "Shaft Inertia Constant [s]"; Vnom "Nominal Voltage [V]"; fan_load "Fan Load"; exciter_param "Exciter Machine Parameters"
      mask help:
      | A generator system block implements a generic power generation unit consisting of a gearbox, a synchronous generator, a synchronous exciter and exciter controls.
      | The generator size can be selected from the drop window below.
      | (For advanced-users) When the User-defined option is selected from the drop window, the generator parameters can be manually specified in the tabs below.
      |
      | Block Inputs:
      |
      | #1: Jet engine low pressure spool [RPM]
      | #2: Exciter system supply voltage [V]
      | #3: Synchronous reference frame line currents  [A]
      |
      | Block Output:
      |
      | #1: Synchronous reference frame line voltages [V]
      | #2: Exciter system supply current [A]
      | #3: Electromagnetic torque on the low pressure spool  [N-M]
      | #4: Heat rejected to the cooling system or ambient [W]
      mask init: same as Boeing787_NewMission_ElectricalThermal/Electrical/Generation Unit Sync-Sync
      mask Help: eval('open(''Generator System_help.html'')');
      mask TypeOptions machine_mode: 20kVA_Gen | 52.5kVA_Gen | 100kVA_Gen | 300kVA_Gen | 800kVA_Gen | 1MVA_Gen | User-defined
      mask Callback machine_mode:
      | h=get_param(gcb,'handle');
      | hblock=get(h);
      | data=load('GenProp.mat');
      | 
      | if strcmp(hblock.machine_mode,'User-defined')==1;
      |     adv_warn=warndlg(sprintf('User-defined parameters may lead to an unstable build.'));
      | 
      |     % grabs current values of enabled GUI parameters
      |     mskenabl = get_param(gcb,'MaskEnables');
      |     mskenabl(1:size(mskenabl,1)) = {'on'};  % sets all parameters to enable
      |     set_param(gcb,'MaskEnables',mskenabl)
      | 
      | else
      |     % For each generator preset references a column from GenProp.mat
      |     if strcmp(hblock.machine_mode,'20kVA_Gen')==1; n=1;
      |     elseif strcmp(hblock.machine_mode,'52.5kVA_Gen')==1; n=2;
      |     elseif strcmp(hblock.machine_mode,'100kVA_Gen')==1; n=3;
      |     elseif strcmp(hblock.machine_mode,'300kVA_Gen')==1; n=4;
      |     elseif strcmp(hblock.machine_mode,'800kVA_Gen')==1; n=5;
      |     elseif strcmp(hblock.machine_mode,'1MVA_Gen')==1; n=6;
      |     end
      |     % Set each parameter of the generator
      |     set1=num2str(data.r(1,n));
      |     set2=num2str(data.r(2,n));
      |     set3=num2str(data.r(3,n));
      |     set4=num2str(data.r(4,n));
      |     set_param(gcb,'Rs',set1,'Xls',set2,'Xmd',set3,'Xmq',set4)
      |     set1=num2str(data.r(5,n));
      |     set2=num2str(data.r(6,n));
      |     set_param(gcb,'R_fd',set1,'Xlfd',set2) %5 and 6
      |     set1=num2str(data.r(7,n));
      |     set2=num2str(data.r(8,n));
      |     set3=num2str(data.r(9,n));
      |     set4=num2str(data.r(10,n));
      |     set5=num2str(data.r(11,n));
      |     set6=num2str(data.r(12,n));
      |     set_param(gcb,'R_1d',set1,'Xl1d',set2,'R_1q',set3,'Xl1q',set4,'R_2q',set5,'Xl2q',set6) %7-12
      |     set1=num2str(data.r(14,n));
      |     set2=num2str(data.r(15,n));
      |     set3=num2str(data.r(16,n));
      |     set_param(gcb,'ws',set1,'RTL',set2,'XTL',set3)
      |     set1=num2str(data.r(17,n));
      |     set2=num2str(data.r(18,n));
      |     set3=num2str(data.r(19,n));
      |     set4=num2str(data.r(20,n));
      |     set5=num2str(data.r(21,n));
      |     set6=num2str(data.r(22,n));
      |     set_param(gcb,'KA',set1,'KF',set2,'T_f',set3,'TA',set4,'KE',set5,'TE',set6)
      |     set1=num2str(data.r(23,n));
      |     set2=num2str(data.r(24,n));
      |     set3=num2str(data.r(25,n));
      |     set4=num2str(data.r(13,n));
      |     set5=num2str(data.r(26,n));
      |     set_param(gcb,'SB',set1,'VBDQ',set2,'wB',set3,'P',set4,'H',set5)
      |     set1=num2str(1/data.r(27,n));
      |     set2=num2str(data.r(28,n));
      |     set_param(gcb,'R_conv_gen',set1,'mc_gen',set2)
      | 
      |     % grabs current values of enabled GUI parameters
      |     mskenabl = get_param(gcb,'MaskEnables');
      |     % sets all parameters to enable
      |     mskenabl(2:size(mskenabl,1)-3) = {'off'};
      |     set_param(gcb,'MaskEnables',mskenabl)
      | 
      | 
      | end
      | 
      | 
      | clear h hblock n data mskenabl
      | clear set1 set2 set3 set4 set5 set6
      mask Display:
      | image(imread('Generator.png')) % Load image
      | 
      | % Define inputs
      | 
      | port_label('input',1,'{\bf \omega_s_h_a_f_t}','Texmode','on')
      | port_label('input',2,'{\bf V_D_C}','Texmode','on')
      | port_label('input',3,'{\bf I_d_q_0}','Texmode','on')
      | port_label('input',4,'{\bf Temp}','Texmode','on')
      | 
      | % Define outputs
      | 
      | port_label('output',1,'{\bf V_d_q_0}','Texmode','on')
      | port_label('output',2,'{\bf I_D_C}','Texmode','on')
      | port_label('output',3,'{\bf \tau}','Texmode','on')
      | port_label('output',4,'{\bf P_l_o_s_s}','Texmode','on')
      | 
      | % % Define inputs
      | %
      | % port_label('input',1,'{\bf Generator Speed}','Texmode','on')
      | % port_label('input',2,'{\bf Battery Voltage}','Texmode','on')
      | % port_label('input',3,'{\bf Line Currents}','Texmode','on')
      | %
      | % % Define outputs
      | %
      | % port_label('output',1,'{\bf Line Voltages}','Texmode','on')
      | % port_label('output',2,'{\bf Battery Current}','Texmode','on')
      | % port_label('output',3,'{\bf Generator Torque}','Texmode','on')
      | % port_label('output',4,'{\bf Power Loss}','Texmode','on')
  Generation Unit Sync-Sync4 : Subsystem  AncestorBlock=PowerFlowLib/Energy & Power Systems/Electrical/Systems/Generation Unit Sync-Sync  mask{machine_mode=300kVA_Gen, Rs=0.007845, Xls=0.0030003, Xmd=0.83467, Xmq=0.0009001, R_fd=0.0024787, Xlfd=0.12144, R_1d=0.072117, Xl1d=0.60648, R_1q=0.019173, R_2q=0.019173, Xl1q=0.10831, Xl2q=0.10831, ws=377, RTL=0.001, XTL=0.1, KA=20, KF=0.063, T_f=0.35, TA=0.2, KE=1, TE=0.314, SB=300000, VBDQ=100, wB=377, P=2, H=0.17945, R_conv_gen=0.05, mc_gen=10000, Vnom=230, fan_load='init_fan_characteristics.mat', exciter_param='exciter.mat'}
      mask prompts: machine_mode "Machine Preset"; Rs "Stator Resistance [ohm]"; Xls "Stator Leakage Reactance [ohm]"; Xmd "Magnetizing Direct Axis Reactance [ohm]"; Xmq "Magnetizing Quadrature Axis Reactance [ohm]"; R_fd "Field Resistance [ohm]"; Xlfd "Field Leakage Reactance [ohm]"; R_1d "Transient Direct Axis Resistance [ohm]"; Xl1d "Transient Leakage Direct Axis Reactance [ohm]"; R_1q "Transient Quadrature Axis Resistance [ohm]"; R_2q "Subtransient Quadrature Axis Resistance [ohm]"; Xl1q "Transient Leakage Quadrature Axis Reactance [ohm]"; Xl2q "Subtransient Leakage Quadrature Axis Reactance [ohm]"; ws "Rotational Speed [rad/s]"; RTL "Resistance [ohm]"; XTL "Reactance [ohm]"; SB "Baes Complex Power [VA]"; VBDQ "Base Direct and Quadrature Axis Armature Voltage [V]"; wB "Base Electrical Frequency [rad/s]"; P "Number of Pole Pairs"; H "Shaft Inertia Constant [s]"; Vnom "Nominal Voltage [V]"; fan_load "Fan Load"; exciter_param "Exciter Machine Parameters"
      mask help:
      | A generator system block implements a generic power generation unit consisting of a gearbox, a synchronous generator, a synchronous exciter and exciter controls.
      | The generator size can be selected from the drop window below.
      | (For advanced-users) When the User-defined option is selected from the drop window, the generator parameters can be manually specified in the tabs below.
      |
      | Block Inputs:
      |
      | #1: Jet engine low pressure spool [RPM]
      | #2: Exciter system supply voltage [V]
      | #3: Synchronous reference frame line currents  [A]
      |
      | Block Output:
      |
      | #1: Synchronous reference frame line voltages [V]
      | #2: Exciter system supply current [A]
      | #3: Electromagnetic torque on the low pressure spool  [N-M]
      | #4: Heat rejected to the cooling system or ambient [W]
      mask init: same as Boeing787_NewMission_ElectricalThermal/Electrical/Generation Unit Sync-Sync
      mask Help: eval('open(''Generator System_help.html'')');
      mask TypeOptions machine_mode: 20kVA_Gen | 52.5kVA_Gen | 100kVA_Gen | 300kVA_Gen | 800kVA_Gen | 1MVA_Gen | User-defined
      mask Callback machine_mode:
      | h=get_param(gcb,'handle');
      | hblock=get(h);
      | data=load('GenProp.mat');
      | 
      | if strcmp(hblock.machine_mode,'User-defined')==1;
      |     adv_warn=warndlg(sprintf('User-defined parameters may lead to an unstable build.'));
      | 
      |     % grabs current values of enabled GUI parameters
      |     mskenabl = get_param(gcb,'MaskEnables');
      |     mskenabl(1:size(mskenabl,1)) = {'on'};  % sets all parameters to enable
      |     set_param(gcb,'MaskEnables',mskenabl)
      | 
      | else
      |     % For each generator preset references a column from GenProp.mat
      |     if strcmp(hblock.machine_mode,'20kVA_Gen')==1; n=1;
      |     elseif strcmp(hblock.machine_mode,'52.5kVA_Gen')==1; n=2;
      |     elseif strcmp(hblock.machine_mode,'100kVA_Gen')==1; n=3;
      |     elseif strcmp(hblock.machine_mode,'300kVA_Gen')==1; n=4;
      |     elseif strcmp(hblock.machine_mode,'800kVA_Gen')==1; n=5;
      |     elseif strcmp(hblock.machine_mode,'1MVA_Gen')==1; n=6;
      |     end
      |     % Set each parameter of the generator
      |     set1=num2str(data.r(1,n));
      |     set2=num2str(data.r(2,n));
      |     set3=num2str(data.r(3,n));
      |     set4=num2str(data.r(4,n));
      |     set_param(gcb,'Rs',set1,'Xls',set2,'Xmd',set3,'Xmq',set4)
      |     set1=num2str(data.r(5,n));
      |     set2=num2str(data.r(6,n));
      |     set_param(gcb,'R_fd',set1,'Xlfd',set2) %5 and 6
      |     set1=num2str(data.r(7,n));
      |     set2=num2str(data.r(8,n));
      |     set3=num2str(data.r(9,n));
      |     set4=num2str(data.r(10,n));
      |     set5=num2str(data.r(11,n));
      |     set6=num2str(data.r(12,n));
      |     set_param(gcb,'R_1d',set1,'Xl1d',set2,'R_1q',set3,'Xl1q',set4,'R_2q',set5,'Xl2q',set6) %7-12
      |     set1=num2str(data.r(14,n));
      |     set2=num2str(data.r(15,n));
      |     set3=num2str(data.r(16,n));
      |     set_param(gcb,'ws',set1,'RTL',set2,'XTL',set3)
      |     set1=num2str(data.r(17,n));
      |     set2=num2str(data.r(18,n));
      |     set3=num2str(data.r(19,n));
      |     set4=num2str(data.r(20,n));
      |     set5=num2str(data.r(21,n));
      |     set6=num2str(data.r(22,n));
      |     set_param(gcb,'KA',set1,'KF',set2,'T_f',set3,'TA',set4,'KE',set5,'TE',set6)
      |     set1=num2str(data.r(23,n));
      |     set2=num2str(data.r(24,n));
      |     set3=num2str(data.r(25,n));
      |     set4=num2str(data.r(13,n));
      |     set5=num2str(data.r(26,n));
      |     set_param(gcb,'SB',set1,'VBDQ',set2,'wB',set3,'P',set4,'H',set5)
      |     set1=num2str(1/data.r(27,n));
      |     set2=num2str(data.r(28,n));
      |     set_param(gcb,'R_conv_gen',set1,'mc_gen',set2)
      | 
      |     % grabs current values of enabled GUI parameters
      |     mskenabl = get_param(gcb,'MaskEnables');
      |     % sets all parameters to enable
      |     mskenabl(2:size(mskenabl,1)-3) = {'off'};
      |     set_param(gcb,'MaskEnables',mskenabl)
      | 
      | 
      | end
      | 
      | 
      | clear h hblock n data mskenabl
      | clear set1 set2 set3 set4 set5 set6
      mask Display:
      | image(imread('Generator.png')) % Load image
      | 
      | % Define inputs
      | 
      | port_label('input',1,'{\bf \omega_s_h_a_f_t}','Texmode','on')
      | port_label('input',2,'{\bf V_D_C}','Texmode','on')
      | port_label('input',3,'{\bf I_d_q_0}','Texmode','on')
      | port_label('input',4,'{\bf Temp}','Texmode','on')
      | 
      | % Define outputs
      | 
      | port_label('output',1,'{\bf V_d_q_0}','Texmode','on')
      | port_label('output',2,'{\bf I_D_C}','Texmode','on')
      | port_label('output',3,'{\bf \tau}','Texmode','on')
      | port_label('output',4,'{\bf P_l_o_s_s}','Texmode','on')
      | 
      | % % Define inputs
      | %
      | % port_label('input',1,'{\bf Generator Speed}','Texmode','on')
      | % port_label('input',2,'{\bf Battery Voltage}','Texmode','on')
      | % port_label('input',3,'{\bf Line Currents}','Texmode','on')
      | %
      | % % Define outputs
      | %
      | % port_label('output',1,'{\bf Line Voltages}','Texmode','on')
      | % port_label('output',2,'{\bf Battery Current}','Texmode','on')
      | % port_label('output',3,'{\bf Generator Torque}','Texmode','on')
      | % port_label('output',4,'{\bf Power Loss}','Texmode','on')
  Generation Unit Sync-Sync5 : Subsystem  AncestorBlock=PowerFlowLib/Energy & Power Systems/Electrical/Systems/Generation Unit Sync-Sync  mask{machine_mode=300kVA_Gen, Rs=0.007845, Xls=0.0030003, Xmd=0.83467, Xmq=0.0009001, R_fd=0.0024787, Xlfd=0.12144, R_1d=0.072117, Xl1d=0.60648, R_1q=0.019173, R_2q=0.019173, Xl1q=0.10831, Xl2q=0.10831, ws=377, RTL=0.001, XTL=0.1, KA=20, KF=0.063, T_f=0.35, TA=0.2, KE=1, TE=0.314, SB=300000, VBDQ=100, wB=377, P=2, H=0.17945, R_conv_gen=0.05, mc_gen=10000, Vnom=230, fan_load='init_fan_characteristics.mat', exciter_param='exciter.mat'}
      mask prompts: machine_mode "Machine Preset"; Rs "Stator Resistance [ohm]"; Xls "Stator Leakage Reactance [ohm]"; Xmd "Magnetizing Direct Axis Reactance [ohm]"; Xmq "Magnetizing Quadrature Axis Reactance [ohm]"; R_fd "Field Resistance [ohm]"; Xlfd "Field Leakage Reactance [ohm]"; R_1d "Transient Direct Axis Resistance [ohm]"; Xl1d "Transient Leakage Direct Axis Reactance [ohm]"; R_1q "Transient Quadrature Axis Resistance [ohm]"; R_2q "Subtransient Quadrature Axis Resistance [ohm]"; Xl1q "Transient Leakage Quadrature Axis Reactance [ohm]"; Xl2q "Subtransient Leakage Quadrature Axis Reactance [ohm]"; ws "Rotational Speed [rad/s]"; RTL "Resistance [ohm]"; XTL "Reactance [ohm]"; SB "Baes Complex Power [VA]"; VBDQ "Base Direct and Quadrature Axis Armature Voltage [V]"; wB "Base Electrical Frequency [rad/s]"; P "Number of Pole Pairs"; H "Shaft Inertia Constant [s]"; Vnom "Nominal Voltage [V]"; fan_load "Fan Load"; exciter_param "Exciter Machine Parameters"
      mask help:
      | A generator system block implements a generic power generation unit consisting of a gearbox, a synchronous generator, a synchronous exciter and exciter controls.
      | The generator size can be selected from the drop window below.
      | (For advanced-users) When the User-defined option is selected from the drop window, the generator parameters can be manually specified in the tabs below.
      |
      | Block Inputs:
      |
      | #1: Jet engine low pressure spool [RPM]
      | #2: Exciter system supply voltage [V]
      | #3: Synchronous reference frame line currents  [A]
      |
      | Block Output:
      |
      | #1: Synchronous reference frame line voltages [V]
      | #2: Exciter system supply current [A]
      | #3: Electromagnetic torque on the low pressure spool  [N-M]
      | #4: Heat rejected to the cooling system or ambient [W]
      mask init: same as Boeing787_NewMission_ElectricalThermal/Electrical/Generation Unit Sync-Sync
      mask Help: eval('open(''Generator System_help.html'')');
      mask TypeOptions machine_mode: 20kVA_Gen | 52.5kVA_Gen | 100kVA_Gen | 300kVA_Gen | 800kVA_Gen | 1MVA_Gen | User-defined
      mask Callback machine_mode:
      | h=get_param(gcb,'handle');
      | hblock=get(h);
      | data=load('GenProp.mat');
      | 
      | if strcmp(hblock.machine_mode,'User-defined')==1;
      |     adv_warn=warndlg(sprintf('User-defined parameters may lead to an unstable build.'));
      | 
      |     % grabs current values of enabled GUI parameters
      |     mskenabl = get_param(gcb,'MaskEnables');
      |     mskenabl(1:size(mskenabl,1)) = {'on'};  % sets all parameters to enable
      |     set_param(gcb,'MaskEnables',mskenabl)
      | 
      | else
      |     % For each generator preset references a column from GenProp.mat
      |     if strcmp(hblock.machine_mode,'20kVA_Gen')==1; n=1;
      |     elseif strcmp(hblock.machine_mode,'52.5kVA_Gen')==1; n=2;
      |     elseif strcmp(hblock.machine_mode,'100kVA_Gen')==1; n=3;
      |     elseif strcmp(hblock.machine_mode,'300kVA_Gen')==1; n=4;
      |     elseif strcmp(hblock.machine_mode,'800kVA_Gen')==1; n=5;
      |     elseif strcmp(hblock.machine_mode,'1MVA_Gen')==1; n=6;
      |     end
      |     % Set each parameter of the generator
      |     set1=num2str(data.r(1,n));
      |     set2=num2str(data.r(2,n));
      |     set3=num2str(data.r(3,n));
      |     set4=num2str(data.r(4,n));
      |     set_param(gcb,'Rs',set1,'Xls',set2,'Xmd',set3,'Xmq',set4)
      |     set1=num2str(data.r(5,n));
      |     set2=num2str(data.r(6,n));
      |     set_param(gcb,'R_fd',set1,'Xlfd',set2) %5 and 6
      |     set1=num2str(data.r(7,n));
      |     set2=num2str(data.r(8,n));
      |     set3=num2str(data.r(9,n));
      |     set4=num2str(data.r(10,n));
      |     set5=num2str(data.r(11,n));
      |     set6=num2str(data.r(12,n));
      |     set_param(gcb,'R_1d',set1,'Xl1d',set2,'R_1q',set3,'Xl1q',set4,'R_2q',set5,'Xl2q',set6) %7-12
      |     set1=num2str(data.r(14,n));
      |     set2=num2str(data.r(15,n));
      |     set3=num2str(data.r(16,n));
      |     set_param(gcb,'ws',set1,'RTL',set2,'XTL',set3)
      |     set1=num2str(data.r(17,n));
      |     set2=num2str(data.r(18,n));
      |     set3=num2str(data.r(19,n));
      |     set4=num2str(data.r(20,n));
      |     set5=num2str(data.r(21,n));
      |     set6=num2str(data.r(22,n));
      |     set_param(gcb,'KA',set1,'KF',set2,'T_f',set3,'TA',set4,'KE',set5,'TE',set6)
      |     set1=num2str(data.r(23,n));
      |     set2=num2str(data.r(24,n));
      |     set3=num2str(data.r(25,n));
      |     set4=num2str(data.r(13,n));
      |     set5=num2str(data.r(26,n));
      |     set_param(gcb,'SB',set1,'VBDQ',set2,'wB',set3,'P',set4,'H',set5)
      |     set1=num2str(1/data.r(27,n));
      |     set2=num2str(data.r(28,n));
      |     set_param(gcb,'R_conv_gen',set1,'mc_gen',set2)
      | 
      |     % grabs current values of enabled GUI parameters
      |     mskenabl = get_param(gcb,'MaskEnables');
      |     % sets all parameters to enable
      |     mskenabl(2:size(mskenabl,1)-3) = {'off'};
      |     set_param(gcb,'MaskEnables',mskenabl)
      | 
      | 
      | end
      | 
      | 
      | clear h hblock n data mskenabl
      | clear set1 set2 set3 set4 set5 set6
      mask Display:
      | image(imread('Generator.png')) % Load image
      | 
      | % Define inputs
      | 
      | port_label('input',1,'{\bf \omega_s_h_a_f_t}','Texmode','on')
      | port_label('input',2,'{\bf V_D_C}','Texmode','on')
      | port_label('input',3,'{\bf I_d_q_0}','Texmode','on')
      | port_label('input',4,'{\bf Temp}','Texmode','on')
      | 
      | % Define outputs
      | 
      | port_label('output',1,'{\bf V_d_q_0}','Texmode','on')
      | port_label('output',2,'{\bf I_D_C}','Texmode','on')
      | port_label('output',3,'{\bf \tau}','Texmode','on')
      | port_label('output',4,'{\bf P_l_o_s_s}','Texmode','on')
      | 
      | % % Define inputs
      | %
      | % port_label('input',1,'{\bf Generator Speed}','Texmode','on')
      | % port_label('input',2,'{\bf Battery Voltage}','Texmode','on')
      | % port_label('input',3,'{\bf Line Currents}','Texmode','on')
      | %
      | % % Define outputs
      | %
      | % port_label('output',1,'{\bf Line Voltages}','Texmode','on')
      | % port_label('output',2,'{\bf Battery Current}','Texmode','on')
      | % port_label('output',3,'{\bf Generator Torque}','Texmode','on')
      | % port_label('output',4,'{\bf Power Loss}','Texmode','on')
  Goto39 : Goto  Commented=on  GotoTag=Battery2_Ploss_W
  Ground1 : Ground
  Ground2 : Ground
  Loads : Subsystem
  Memory{1,5..8,10..11} (7 alike) : Memory
  Memory29 : Memory  Commented=on
  Memory32 : Memory  Commented=on
  Mux : Mux
  Mux1 : Mux  Inputs=2
  Mux2 : Mux  Inputs=2
  Mux4 : Mux  Inputs=7
  Outputs : Subsystem
  Product{,1..9} (10 alike) : Product
  Sum3 : Sum  Inputs=++++
  Terminator : Terminator
  Terminator3 : Terminator
  Terminator6 : Terminator
  Thermal Interface : Subsystem
  To Workspace : ToWorkspace  VariableName=Gen1Power_W  SaveFormat=Structure With Time  SampleTime=-1
  To Workspace1 : ToWorkspace  VariableName=APU2Power_W  SaveFormat=Structure With Time  SampleTime=-1
  To Workspace10 : ToWorkspace  VariableName=dc28  SaveFormat=Structure With Time  SampleTime=0.1
  To Workspace11 : ToWorkspace  VariableName=ac115  SaveFormat=Structure With Time  SampleTime=0.1
  To Workspace2 : ToWorkspace  VariableName=Gen3Power_W  SaveFormat=Structure With Time  SampleTime=-1
  To Workspace3 : ToWorkspace  VariableName=totalacload  SaveFormat=Timeseries  SampleTime=-1
  To Workspace4 : ToWorkspace  VariableName=totaldcload  SaveFormat=Timeseries  SampleTime=-1
  To Workspace5 : ToWorkspace  VariableName=Gen2Power_W  SaveFormat=Structure With Time  SampleTime=-1
  To Workspace6 : ToWorkspace  VariableName=Gen4Power_W  SaveFormat=Structure With Time  SampleTime=-1
  To Workspace7 : ToWorkspace  VariableName=APU1Power_W  SaveFormat=Structure With Time  SampleTime=-1
  To Workspace8 : ToWorkspace  VariableName=ac230  SaveFormat=Structure With Time  SampleTime=0.1
  To Workspace9 : ToWorkspace  VariableName=dc270  SaveFormat=Structure With Time  SampleTime=0.1
  Transformer-rectifier : Subsystem  AncestorBlock=PowerFlowLib/Energy & Power Systems/Electrical/Systems/Transformer-rectifier  mask{pu=1}
      mask prompts: pu "Voltage Regulation Level (p.u.)"
      mask Display:
      | image('TRU.png')
      | % Define Inputs
      | port_label('input',1,'{\bf V_d_q_0}','Texmode','on')
      | port_label('input',2,'{\bf i_{DC}}','Texmode','on')
      | 
      | % Define Outputs
      | port_label('output',1,'{\bf V_D_C}','Texmode','on')
      | port_label('output',2,'{\bf I_d_q_0}','Texmode','on')
      | 
      | 
      | % % Define Inputs
      | % port_label('input',1,'{\bf Line Voltage}','Texmode','on')
      | % port_label('input',2,'{\bf Line Voltage}','Texmode','on')
      | %
      | % % Define Outputs
      | % port_label('output',1,'{\bf Line Voltage}','Texmode','on')
      | % port_label('output',2,'{\bf Line Voltage}','Texmode','on')
  Transformer-rectifier1 : Subsystem  AncestorBlock=PowerFlowLib/Energy & Power Systems/Electrical/Systems/Transformer-rectifier  mask{pu=1}
      mask prompts: pu "Voltage Regulation Level (p.u.)"
      mask Display:
      | image('TRU.png')
      | % Define Inputs
      | port_label('input',1,'{\bf V_d_q_0}','Texmode','on')
      | port_label('input',2,'{\bf i_{DC}}','Texmode','on')
      | 
      | % Define Outputs
      | port_label('output',1,'{\bf V_D_C}','Texmode','on')
      | port_label('output',2,'{\bf I_d_q_0}','Texmode','on')
      | 
      | 
      | % % Define Inputs
      | % port_label('input',1,'{\bf Line Voltage}','Texmode','on')
      | % port_label('input',2,'{\bf Line Voltage}','Texmode','on')
      | %
      | % % Define Outputs
      | % port_label('output',1,'{\bf Line Voltage}','Texmode','on')
      | % port_label('output',2,'{\bf Line Voltage}','Texmode','on')
  Vector Concatenate{,1..3} (4 alike) : Concatenate  NumInputs=1  Mode=Multidimensional array  ConcatenateDimension=2
  Vector Concatenate4 : Concatenate  Mode=Multidimensional array  ConcatenateDimension=2
  Vector Concatenate5 : Concatenate  Mode=Multidimensional array  ConcatenateDimension=2
  Vector Concatenate7 : Concatenate  Commented=on  Mode=Multidimensional array  ConcatenateDimension=2
  ELEC : Outport
  tag scope: AC115_Power=global, AC230_Power=global, AC_115V_Bus=global, APU_Torque_Nm=global, DC270_Power=global, DC28_Power=global, DC_270V_Bus=global, DC_28V_Bus=global, Gen_Bus1=global, Gen_Bus2=global, Idq0_230AC=global, Idq0_ATRU=global, Idq0_ATU=global, Idq0_TRU=global, enable2=global, enable=global
  wires:
  230 Vac Distr/1(Vbus1) -> Transformer-rectifier/1(vqd0), Product3/1, To Workspace8/1, Enabled_AC_Loadloss/2(Vdq0)
  230 Vac Distr/2(Vbus2) -> Transformer-rectifier1/1(vqd0), Auto Transformer/1(vqd0)
  [enable] -> Enabled_AC_Loadloss/Enable
  DC Bus 1/1(Vbus) -> Enabled DC Load1/1(VDC), Product/2
  DC Bus 3/1(Vbus) -> Product2/1, Enabled DC Load2/1
  Enabled DC Load2/1 -> Product2/2, DC Bus 3/4(Load current)
  [enable2] -> Enabled DC Load1/Enable
  [enable] -> Enabled_AC_Loadloss1/Enable
  [enable] -> Enabled DC Load2/Enable
  Enabled_AC_Loadloss1/1 -> Auto Transformer/2(iAC), Product1/1
  Memory32/1 -> BATTERY/1
  1-dim8/1 -> Memory32/1
  From22/1 -> Vector Concatenate7/1
  From25/1 -> Vector Concatenate7/2
  Vector Concatenate7/1 -> 1-dim8/1
  Memory29/1 -> BATTERY/2
  From59/1 -> Memory29/1
  [AC_230V_Load] -> Enabled_AC_Loadloss/1(Load Master Vector)
  Enabled_AC_Loadloss/2(loss) -> [loadloss_1]
  Add/1 -> To Workspace4/1
  Add1/1 -> To Workspace3/1
  Enabled_AC_Loadloss1/2 -> [loadloss_2]
  [AC_115V_Load] -> Enabled_AC_Loadloss1/1
  [DC_270V_Load] -> Enabled DC Load1/2(Control)
  [DC_270V_Bus] -> DC Bus 1/1(Select)
  [DC_28V_Bus] -> DC Bus 3/1(Select)
  BATTERY/2 -> Goto39/1
  [Left_Wing_SCVGU_Torque_Nm] -> Outputs/1(Left_Wing_Toqrue_Nm)
  [Right_Wing_SCVGU_Torque_Nm] -> Outputs/2(Rght_Wing_Torque_Nm)
  [APU_Torque_Nm] -> Outputs/3(APU_Torque_Nm)
  [DC_28V_Load] -> Enabled DC Load2/2
  DC Bus 1/3(IDC_2) -> Terminator3/1
  DC Bus 1/2(IDC_1) -> Transformer-rectifier/2(iDC)
  DC Bus 3/2(IDC_1) -> Transformer-rectifier1/2(iDC)
  DC Bus 3/3(IDC_2) -> Terminator6/1
  Transformer-rectifier1/1(vout) -> To Workspace10/1
  Outputs/1(Electrical) -> ELEC/1
  Constant1/1 -> DC Bus 1/2(VDC_1)
  Product3/1 -> [AC230_Power]
  [AC230_Power] -> Add1/1
  Product/1 -> [DC270_Power]
  Product1/1 -> [AC115_Power]
  [AC115_Power] -> Add1/2
  [DC270_Power] -> Add/1
  [DC28_Power] -> Add/2
  Constant/1 -> DC Bus 3/2(VDC_1)
  First-Order Filter/1 -> 230 Vac Distr/7(I_Bus)
  [DC_270_Voltage] -> Outputs/4(DC_Voltage_270)
  ECS/1 -> Terminator/1
  Enabled_AC_Loadloss/1(Idq0) -> [Idq0_230AC]
  [Idq0_230AC] -> Product3/2
  Transformer-rectifier/2(iqd0) -> [Idq0_ATRU]
  Enabled DC Load1/1(iDC) -> Product/1, [iDC270V]
  Auto Transformer/2(iqd0) -> [Idq0_ATU]
  Auto Transformer/1(vout) -> Enabled_AC_Loadloss1/2, To Workspace11/1, Product1/2
  Transformer-rectifier1/2(iqd0) -> [Idq0_TRU]
  [Idq0_230AC] -> Sum3/1
  [Idq0_ATRU] -> Sum3/2
  [Idq0_ATU] -> Sum3/3
  [Idq0_TRU] -> Sum3/4
  Constant2/1 -> [Eng1_Spool_RPM], [Eng2_Spool_RPM]
  Add3/1 -> [Right_Wing_SCVGU_Torque_Nm]
  " "/1 -> [Left_Wing_SCVGU_Torque_Nm]
  [Gen_1_Torque_Nm] -> Add3/1
  [Gen_2_Torque_Nm] -> Add3/2
  [Gen_3_Torque_Nm] -> " "/1
  [Gen_4_Torque_Nm] -> " "/2
  " 1"/1 -> [APU_Torque_Nm]
  [APU_1_Torque_Nm] -> " 1"/1
  [APU_2_Torque_Nm] -> " 1"/2
  [Battery2_Ploss_W] -> Thermal Interface/3(Battery Loss [1])
  Mux2/1 -> Thermal Interface/4(Loadloss_W)
  [loadloss_1] -> Mux2/1
  [loadloss_2] -> Mux2/2
  [APU_2_Ploss_W] -> Mux1/2
  [APU_1_Ploss_W] -> Mux1/1
  [Gen_1_Ploss_W] -> Mux/1
  [Gen_2_Ploss_W] -> Mux/2
  [Gen_3_Ploss_W] -> Mux/3
  [Gen_4_Ploss_W] -> Mux/4
  Mux/1 -> Thermal Interface/1(Generator Loss [4])
  Mux1/1 -> Thermal Interface/2(APU Loss [2])
  Thermal Interface/1(Tgen1) -> [Gen1_Temp]
  Thermal Interface/2(Tgen2) -> [Gen2_Temp]
  Thermal Interface/3(Tgen3) -> [Gen3_Temp]
  Thermal Interface/4(Tgen4) -> [Gen4_Temp]
  Thermal Interface/5(Tgen5) -> [Gen5_Temp]
  Thermal Interface/6(Tgen6) -> [Gen6_Temp]
  Bus Controls/1(Gen_Bus1) -> [Gen_Bus1]
  Bus Controls/2(Gen_Bus2) -> [Gen_Bus2]
  Bus Controls/5(28V_DC_Bus) -> [DC_28V_Bus]
  Bus Controls/4(115V_AC_Bus) -> [AC_115V_Bus]
  Bus Controls/3(270V_DC_Bus) -> [DC_270V_Bus]
  Loads/1(230 Vac Loads) -> [AC_230V_Load]
  Loads/2(115 Vac Loads) -> [AC_115V_Load]
  Loads/3(270 Vdc Loads) -> [DC_270V_Load]
  Loads/4(28 Vdc Loads) -> [DC_28V_Load]
  Enable time 1/1 -> [enable]
  Enable time 2/1 -> [enable2]
  Generation Unit Sync-Sync/1(vdq0) -> 230 Vac Distr/1(Gen 1), Product5/1
  Generation Unit Sync-Sync1/1(vdq0) -> 230 Vac Distr/2(Gen 2), Product7/1
  Generation Unit Sync-Sync2/1(vdq0) -> 230 Vac Distr/3(Gen 3), Product6/1
  Generation Unit Sync-Sync3/1(vdq0) -> 230 Vac Distr/4(Gen 4), Product8/1
  Generation Unit Sync-Sync4/1(vdq0) -> 230 Vac Distr/5(Gen 5), Product9/1
  Generation Unit Sync-Sync5/1(vdq0) -> 230 Vac Distr/6(Gen 6), Product4/1
  [i_MAIN2] -> Memory6/1
  [i_MAIN2] -> Memory7/1
  [i_MAIN1] -> Memory5/1
  Memory7/1 -> Vector Concatenate3/1
  Vector Concatenate3/1 -> 1-dim3/1
  1-dim3/1 -> Generation Unit Sync-Sync3/3(idq0), Product8/2
  Memory6/1 -> Vector Concatenate2/1
  Vector Concatenate2/1 -> 1-dim2/1
  Memory5/1 -> Vector Concatenate1/1
  Vector Concatenate1/1 -> 1-dim1/1
  1-dim1/1 -> Generation Unit Sync-Sync1/3(idq0), Product7/2
  [i_MAIN1] -> Vector Concatenate/1
  Vector Concatenate/1 -> 1-dim/1
  1-dim/1 -> Generation Unit Sync-Sync/3(idq0), Product5/2
  [Eng1_Spool_RPM] -> Generation Unit Sync-Sync/1(engine speed)
  [Gen1_Temp] -> Generation Unit Sync-Sync/4(Temperature)
  Product4/1 -> Gain9/1
  Gain9/1 -> To Workspace1/1
  Vector Concatenate5/1 -> 1-dim5/1
  [i_APU2] -> Memory11/1
  [i_APU1] -> Memory10/1
  Memory10/1 -> Vector Concatenate5/1
  Memory11/1 -> Vector Concatenate5/2
  Product5/1 -> Gain4/1
  Product6/1 -> Gain6/1
  Gain6/1 -> To Workspace2/1
  Product7/1 -> Gain5/1
  Gain5/1 -> To Workspace5/1
  Product8/1 -> Gain7/1
  Gain7/1 -> To Workspace6/1
  Product9/1 -> Gain8/1
  Gain8/1 -> To Workspace7/1
  Generation Unit Sync-Sync4/3(engine torque) -> [APU_1_Torque_Nm]
  Generation Unit Sync-Sync5/3(engine torque) -> [APU_2_Torque_Nm]
  Generation Unit Sync-Sync4/4(Ploss) -> [APU_1_Ploss_W]
  Generation Unit Sync-Sync/4(Ploss) -> [Gen_1_Ploss_W]
  Generation Unit Sync-Sync/3(engine torque) -> [Gen_1_Torque_Nm]
  Generation Unit Sync-Sync1/3(engine torque) -> [Gen_2_Torque_Nm]
  Generation Unit Sync-Sync3/4(Ploss) -> [Gen_4_Ploss_W]
  Generation Unit Sync-Sync2/4(Ploss) -> [Gen_3_Ploss_W]
  Generation Unit Sync-Sync3/3(engine torque) -> [Gen_4_Torque_Nm]
  Generation Unit Sync-Sync2/3(engine torque) -> [Gen_3_Torque_Nm]
  1-dim5/1 -> Gain/1
  Gain/1 -> Generation Unit Sync-Sync4/3(idq0), Product9/2
  Gain1/1 -> Generation Unit Sync-Sync5/3(idq0), Product4/2
  [Eng1_Spool_RPM] -> Generation Unit Sync-Sync1/1(engine speed)
  [Gen2_Temp] -> Generation Unit Sync-Sync1/4(Temperature)
  [Eng2_Spool_RPM] -> Generation Unit Sync-Sync2/1(engine speed)
  [Gen3_Temp] -> Generation Unit Sync-Sync2/4(Temperature)
  [Eng2_Spool_RPM] -> Generation Unit Sync-Sync3/1(engine speed)
  [Gen4_Temp] -> Generation Unit Sync-Sync3/4(Temperature)
  Generation Unit Sync-Sync5/4(Ploss) -> [APU_2_Ploss_W]
  [Eng1_Spool_RPM] -> Gain2/1
  Gain2/1 -> Generation Unit Sync-Sync4/1(engine speed)
  Vector Concatenate4/1 -> 1-dim4/1
  [i_APU2] -> Memory8/1
  [i_APU1] -> Memory1/1
  Memory1/1 -> Vector Concatenate4/1
  Memory8/1 -> Vector Concatenate4/2
  1-dim4/1 -> Gain1/1
  [Eng2_Spool_RPM] -> Gain3/1
  Gain3/1 -> Generation Unit Sync-Sync5/1(engine speed)
  [Gen5_Temp] -> Generation Unit Sync-Sync4/4(Temperature)
  [Gen6_Temp] -> Generation Unit Sync-Sync5/4(Temperature)
  Generation Unit Sync-Sync1/4(Ploss) -> [Gen_2_Ploss_W]
  1-dim2/1 -> Generation Unit Sync-Sync2/3(idq0), Product6/2
  [Bus_28V] -> Generation Unit Sync-Sync5/2(battery voltage)
  [Bus_28V] -> Generation Unit Sync-Sync4/2(battery voltage)
  [Bus_28V] -> Generation Unit Sync-Sync2/2(battery voltage)
  [Bus_28V] -> Generation Unit Sync-Sync3/2(battery voltage)
  [Bus_28V] -> Generation Unit Sync-Sync1/2(battery voltage)
  [Bus_28V] -> Generation Unit Sync-Sync/2(battery voltage)
  Generation Unit Sync-Sync/2(battery current) -> [Gen1_iDC]
  Generation Unit Sync-Sync5/2(battery current) -> [Gen6_iDC]
  Generation Unit Sync-Sync1/2(battery current) -> [Gen2_iDC]
  Generation Unit Sync-Sync2/2(battery current) -> [Gen3_iDC]
  Generation Unit Sync-Sync3/2(battery current) -> [Gen4_iDC]
  Generation Unit Sync-Sync4/2(battery current) -> [Gen5_iDC]
  Gain4/1 -> To Workspace/1
  Sum3/1 -> First-Order Filter/1
  Transformer-rectifier/1(vout) -> To Workspace9/1, [DC_270_Voltage]
  Ground1/1 -> DC Bus 1/3(VDC_2)
  [Gen1_iDC] -> Mux4/2
  [Gen2_iDC] -> Mux4/3
  [Gen3_iDC] -> Mux4/4
  [Gen4_iDC] -> Mux4/5
  [Gen5_iDC] -> Mux4/6
  [Gen6_iDC] -> Mux4/7
  Mux4/1 -> DC Bus 1/4(Load current)
  [iDC270V] -> Mux4/1
  Product2/1 -> [DC28_Power]
  Ground2/1 -> DC Bus 3/3(VDC_2)
  Constant3/1 -> [Bus_28V]
  Eng1/1 -> Bus Selector/1
  Eng2/1 -> Bus Selector1/1
